simulink model "reclaim_product_control"  (R2024a)
settings: Solver=VariableStepAuto  StartTime=0.0  StopTime=10.0  RelTol=1e-3
settings Model: Creator=shadysiam  LastModifiedBy=shadysiam

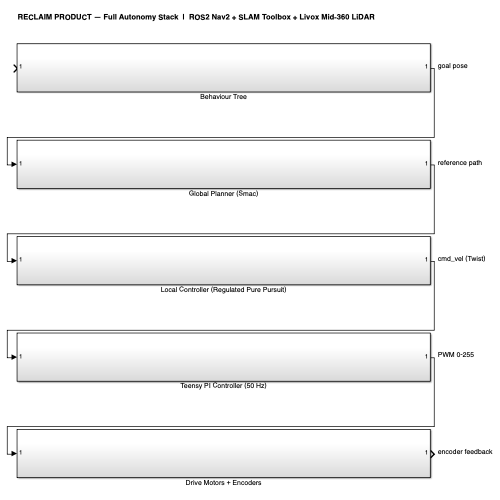
[thumbnail: Simulink's stored preview of the top-level diagram]
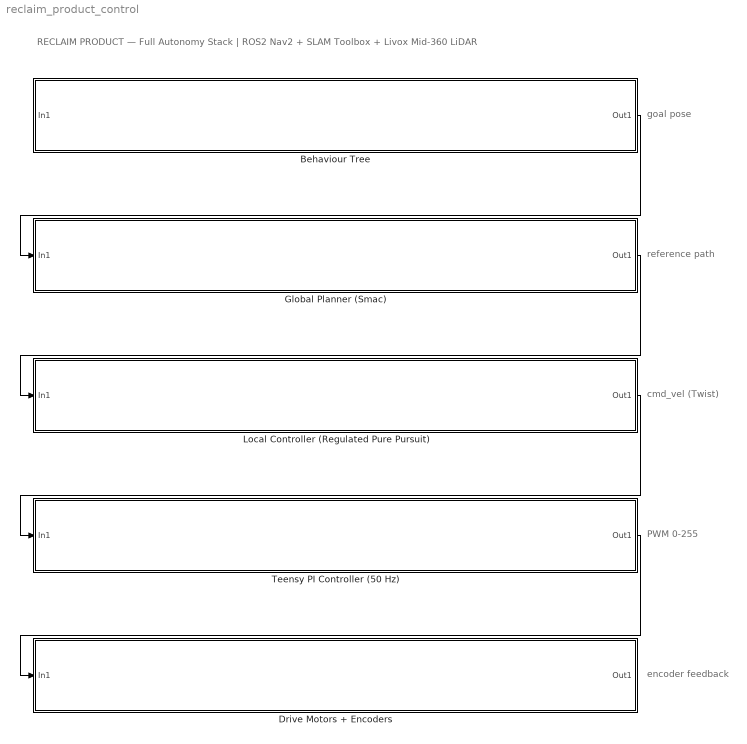
== system reclaim_product_control ==
  note: goal pose
  note: reference path
  note: cmd_vel (Twist)
  note: PWM 0-255
  note: encoder feedback
  note: RECLAIM PRODUCT — Full Autonomy Stack | ROS2 Nav2 + SLAM Toolbox + Livox Mid-360 LiDAR
  Behaviour Tree : Subsystem
  Drive Motors + Encoders : Subsystem
  Global Planner (Smac) : Subsystem
  Local Controller (Regulated Pure Pursuit) : Subsystem
  Teensy PI Controller (50 Hz) : Subsystem
  wires:
  Behaviour Tree/1(Out1) -> Global Planner (Smac)/1(In1)
  Global Planner (Smac)/1(Out1) -> Local Controller (Regulated Pure Pursuit)/1(In1)
  Local Controller (Regulated Pure Pursuit)/1(Out1) -> Teensy PI Controller (50 Hz)/1(In1)
  Teensy PI Controller (50 Hz)/1(Out1) -> Drive Motors + Encoders/1(In1)

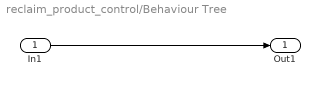
== system reclaim_product_control/Behaviour Tree ==
  In1 : Inport
  Out1 : Outport
  wires:
  In1/1 -> Out1/1

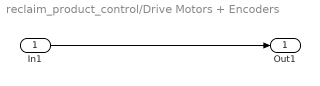
== system reclaim_product_control/Drive Motors + Encoders ==
  In1 : Inport
  Out1 : Outport
  wires:
  In1/1 -> Out1/1

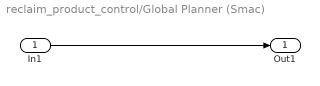
== system reclaim_product_control/Global Planner (Smac) ==
  In1 : Inport
  Out1 : Outport
  wires:
  In1/1 -> Out1/1

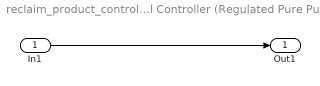
== system reclaim_product_control/Local Controller (Regulated Pure Pursuit) ==
  In1 : Inport
  Out1 : Outport
  wires:
  In1/1 -> Out1/1

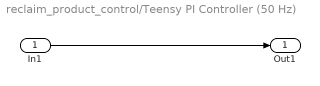
== system reclaim_product_control/Teensy PI Controller (50 Hz) ==
  In1 : Inport
  Out1 : Outport
  wires:
  In1/1 -> Out1/1
